simulink model "Helicoptero_2DOF_EKFv2"  (R2024b)
settings: Solver=FixedStepAuto  StartTime=0.0  StopTime=10  FixedStep=0.001  RelTol=1e-3
values from neighbouring files (symbols this model uses):
  theta_0 = -40.5*pi/180    (= -0.706858347058)    [setup_heli_2d_base.m]
  VMAX_UPM_P = 24    [setup_heli_2d_base.m]
  VMAX_UPM_Y = 15    [setup_heli_2d_base.m]
undefined symbols (not defined in the file or in its folder): B_p, B_y, g, J_eq_p, J_eq_y, K_pp, K_py, K_yp, K_yy, l_cm, m_heli
libraries: simulink x3
settings Model: Creator=david  LastModifiedBy=Usuario

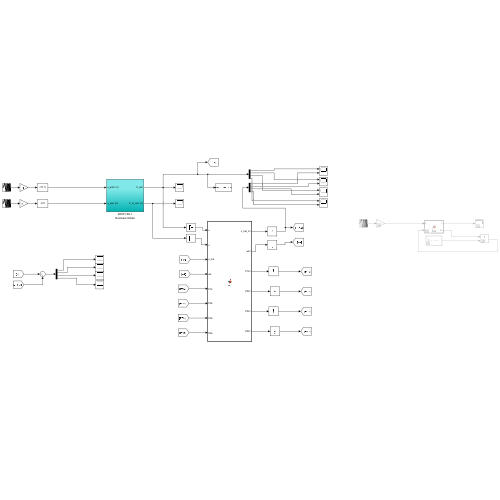
[thumbnail: Simulink's stored preview of the top-level diagram]
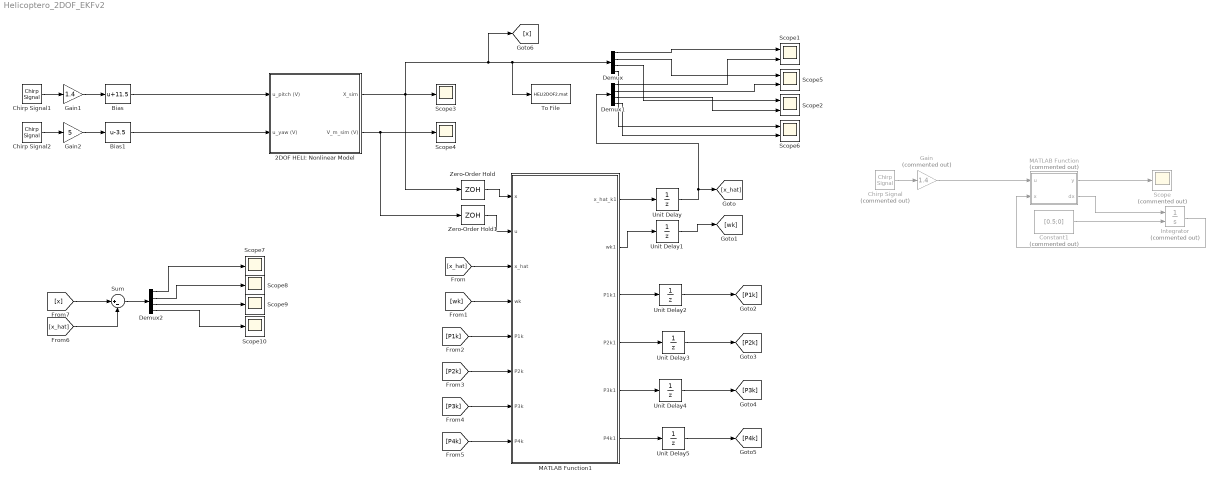
== system Helicoptero_2DOF_EKFv2 ==
  2DOF HELI: Nonlinear Model : Subsystem
  Bias : Bias  Bias=11.5  SaturateOnIntegerOverflow=off
  Bias1 : Bias  Bias=-3.5  SaturateOnIntegerOverflow=off
  Chirp Signal : simulink/Sources/Chirp Signal  Commented=on  f1=0.08  T=10  f2=1
  Chirp Signal1 : simulink/Sources/Chirp Signal  f1=0.08  T=10  f2=1
  Chirp Signal2 : simulink/Sources/Chirp Signal  f1=0.05  T=100  f2=1
  Constant1 : Constant  Commented=on  Value=[0.5;0]
  Demux : Demux
  Demux1 : Demux
  Demux2 : Demux
  Gain : Gain  Commented=on  Gain=1.4
  Gain1 : Gain  Gain=1.4
  Gain2 : Gain  Gain=5
  Integrator : Integrator  Commented=on  InitialConditionSource=external
  MATLAB Function : MATLAB Function  Commented=on  TreatAsAtomicUnit=on
  MATLAB Function1 : MATLAB Function  TreatAsAtomicUnit=on
  Scope : Scope  Commented=on
  Scope{1..2,5..6} (4 alike) : Scope  NumInputPorts=2
  Scope{3..4,7..10} (6 alike) : Scope
  Sum : Sum  Inputs=|+-
  To File : ToFile  Filename=HELI2DOF2.mat  MatrixName=out
  Unit Delay : UnitDelay  SampleTime=-1  HasFrameUpgradeWarning=on
  Unit Delay1 : UnitDelay  InitialCondition=[rand(1,8)]  SampleTime=-1  HasFrameUpgradeWarning=on
  Unit Delay{2..5} (4 alike) : UnitDelay  InitialCondition=eye(2)*50000  SampleTime=-1  HasFrameUpgradeWarning=on
  Zero-Order Hold : ZeroOrderHold  SampleTime=-1
  Zero-Order Hold1 : ZeroOrderHold  SampleTime=-1
  wires:
  MATLAB Function/2(dx) -> Integrator/1
  Integrator/1 -> MATLAB Function/2(x)
  Constant1/1 -> Integrator/2
  MATLAB Function/1(y) -> Scope/1
  Chirp Signal/1 -> Gain/1
  Gain/1 -> MATLAB Function/1(u)
  [P2k] -> MATLAB Function1/6(P2k)
  [P1k] -> MATLAB Function1/5(P1k)
  [wk] -> MATLAB Function1/4(wk)
  [x_hat] -> MATLAB Function1/3(x_hat)
  Demux/1 -> Scope1/1
  Demux/2 -> Scope5/1
  Demux1/1 -> Scope1/2
  Demux1/2 -> Scope5/2
  Unit Delay/1 -> Demux1/1, [x_hat]
  Unit Delay1/1 -> [wk]
  Unit Delay2/1 -> [P1k]
  Unit Delay3/1 -> [P2k]
  MATLAB Function1/1(x_hat_k1) -> Unit Delay/1
  MATLAB Function1/4(P2k1) -> Unit Delay3/1
  MATLAB Function1/3(P1k1) -> Unit Delay2/1
  MATLAB Function1/2(wk1) -> Unit Delay1/1
  Zero-Order Hold/1 -> MATLAB Function1/1(x)
  Zero-Order Hold1/1 -> MATLAB Function1/2(u)
  [P4k] -> MATLAB Function1/8(P4k)
  [P3k] -> MATLAB Function1/7(P3k)
  MATLAB Function1/5(P3k1) -> Unit Delay4/1
  Unit Delay4/1 -> [P3k]
  Unit Delay5/1 -> [P4k]
  MATLAB Function1/6(P4k1) -> Unit Delay5/1
  Gain1/1 -> Bias/1
  Chirp Signal2/1 -> Gain2/1
  Bias1/1 -> 2DOF HELI: Nonlinear Model/2(u_yaw (V))
  Chirp Signal1/1 -> Gain1/1
  Gain2/1 -> Bias1/1
  2DOF HELI: Nonlinear Model/2(V_m_sim (V)) -> Zero-Order Hold1/1, Scope4/1
  Bias/1 -> 2DOF HELI: Nonlinear Model/1(u_pitch (V))
  2DOF HELI: Nonlinear Model/1(X_sim) -> [x], To File/1, Demux/1, Zero-Order Hold/1, Scope3/1
  Demux/3 -> Scope2/1
  Demux1/3 -> Scope2/2
  Demux/4 -> Scope6/1
  Demux1/4 -> Scope6/2
  [x] -> Sum/1
  [x_hat] -> Sum/2
  Sum/1 -> Demux2/1
  Demux2/1 -> Scope7/1
  Demux2/2 -> Scope8/1
  Demux2/3 -> Scope9/1
  Demux2/4 -> Scope10/1

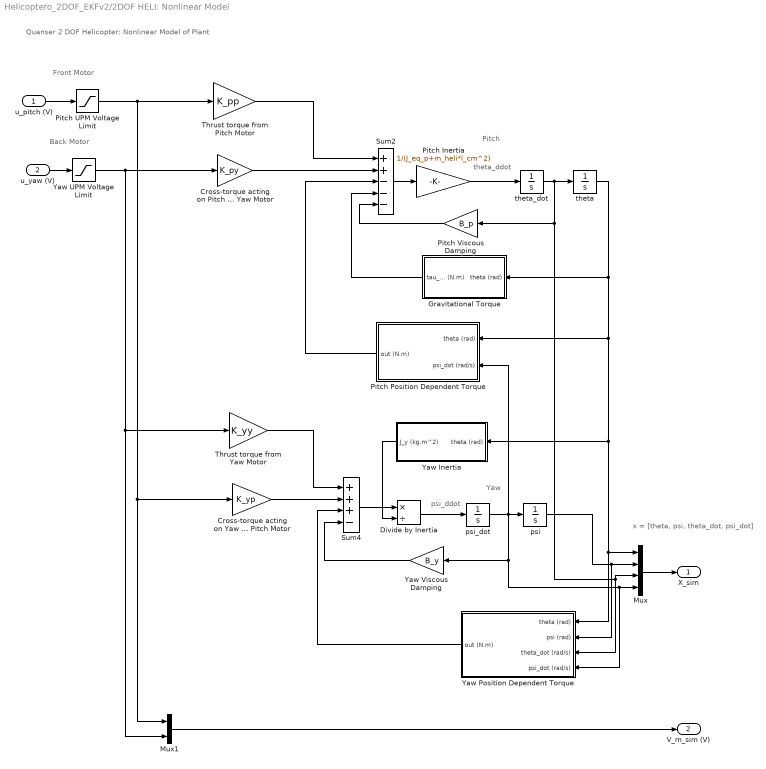
== system Helicoptero_2DOF_EKFv2/2DOF HELI: Nonlinear Model ==
  note: Back Motor
  note: Front Motor
  note: x = [theta, psi, theta_dot, psi_dot]
  note: Quanser 2 DOF Helicopter: Nonlinear Model of Plant
  note: theta_ddot
  note: psi_ddot
  note: Pitch
  note: Yaw
  u_pitch (V) : Inport
  u_yaw (V) : Inport  Port=2
  Cross-torque acting on Pitch from Yaw Motor : Gain  Gain=K_py
  Cross-torque acting on Yaw from Pitch Motor : Gain  Gain=K_yp
  Divide by Inertia : Product  Inputs=*/
  Gravitational Torque : Subsystem
  Mux : Mux
  Mux1 : Mux  Inputs=2
  Pitch Inertia : Gain  Gain=1/(J_eq_p+m_heli*l_cm^2)
  Pitch Position Dependent Torque : Subsystem  AncestorBlock=heli_2d_lib/2DOF Helicopter: Nonlinear Model/Yaw Nonlinear Element
  Pitch UPM Voltage Limit : Saturate  UpperLimit=VMAX_UPM_P  LowerLimit=- VMAX_UPM_P
  Pitch Viscous Damping : Gain  Gain=B_p
  Sum2 : Sum  Inputs=++---
  Sum4 : Sum  Inputs=+++-
  Thrust torque from Pitch Motor : Gain  Gain=K_pp
  Thrust torque from Yaw Motor : Gain  Gain=K_yy
  Yaw Inertia : Subsystem
  Yaw Position Dependent Torque : Subsystem
  Yaw UPM Voltage Limit : Saturate  UpperLimit=VMAX_UPM_Y  LowerLimit=- VMAX_UPM_Y
  Yaw Viscous Damping : Gain  Gain=B_y
  psi : Integrator
  psi_dot : Integrator
  theta : Integrator  InitialCondition=theta_0  LimitOutput=on  UpperSaturationLimit=40.5*pi/180  LowerSaturationLimit=-40.5*pi/180
  theta_dot : Integrator
  X_sim : Outport
  V_m_sim (V) : Outport  Port=2
  wires:
  Pitch Position Dependent Torque/1(out (N.m)) -> Sum2/3
  Gravitational Torque/1(tau_g (N.m)) -> Sum2/4
  Pitch Viscous Damping/1 -> Sum2/5
  Cross-torque acting on Pitch from Yaw Motor/1 -> Sum2/2
  Thrust torque from Pitch Motor/1 -> Sum2/1
  Yaw Inertia/1(J_y (kg.m^2)) -> Divide by Inertia/2
  Divide by Inertia/1 -> psi_dot/1
  Sum4/1 -> Divide by Inertia/1
  Yaw Position Dependent Torque/1(out (N.m)) -> Sum4/3
  Yaw Viscous Damping/1 -> Sum4/4
  psi/1 -> Yaw Position Dependent Torque/2(psi (rad)), Mux/2
  Mux1/1 -> V_m_sim (V)/1
  Yaw UPM Voltage Limit/1 -> Thrust torque from Yaw Motor/1, Mux1/2, Cross-torque acting on Pitch from Yaw Motor/1
  Pitch UPM Voltage Limit/1 -> Mux1/1, Cross-torque acting on Yaw from Pitch Motor/1, Thrust torque from Pitch Motor/1
  Mux/1 -> X_sim/1
  theta/1 -> Gravitational Torque/1(theta (rad)), Pitch Position Dependent Torque/1(theta (rad)), Yaw Position Dependent Torque/1(theta (rad)), Mux/1, Yaw Inertia/1(theta (rad))
  Sum2/1 -> Pitch Inertia/1
  Pitch Inertia/1 -> theta_dot/1
  theta_dot/1 -> Pitch Viscous Damping/1, Yaw Position Dependent Torque/3(theta_dot (rad/s)), Mux/3, theta/1
  Thrust torque from Yaw Motor/1 -> Sum4/1
  Cross-torque acting on Yaw from Pitch Motor/1 -> Sum4/2
  psi_dot/1 -> Yaw Viscous Damping/1, Yaw Position Dependent Torque/4(psi_dot (rad/s)), Mux/4, Pitch Position Dependent Torque/2(psi_dot (rad/s)), psi/1
  u_pitch (V)/1 -> Pitch UPM Voltage Limit/1
  u_yaw (V)/1 -> Yaw UPM Voltage Limit/1

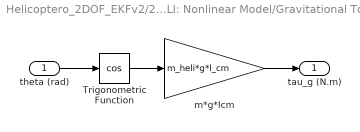
== system Helicoptero_2DOF_EKFv2/2DOF HELI: Nonlinear Model/Gravitational Torque ==
  theta (rad) : Inport
  Trigonometric Function : Trigonometry  Operator=cos  OutputSignalType=real
  m*g*lcm : Gain  Gain=m_heli*g*l_cm
  tau_g (N.m) : Outport
  wires:
  m*g*lcm/1 -> tau_g (N.m)/1
  theta (rad)/1 -> Trigonometric Function/1
  Trigonometric Function/1 -> m*g*lcm/1

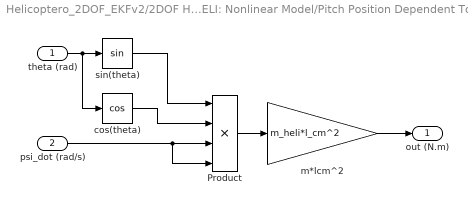
== system Helicoptero_2DOF_EKFv2/2DOF HELI: Nonlinear Model/Pitch Position Dependent Torque ==
  theta (rad) : Inport
  psi_dot (rad/s) : Inport  Port=2
  Product : Product  Inputs=4  RndMeth=Zero
  cos(theta) : Trigonometry  Operator=cos  OutputSignalType=real
  m*lcm^2 : Gain  Gain=m_heli*l_cm^2
  sin(theta) : Trigonometry  OutputSignalType=real
  out (N.m) : Outport
  wires:
  psi_dot (rad/s)/1 -> Product/4, Product/3
  theta (rad)/1 -> cos(theta)/1, sin(theta)/1
  Product/1 -> m*lcm^2/1
  sin(theta)/1 -> Product/1
  cos(theta)/1 -> Product/2
  m*lcm^2/1 -> out (N.m)/1

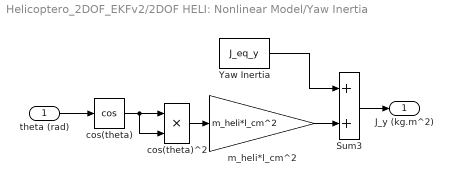
== system Helicoptero_2DOF_EKFv2/2DOF HELI: Nonlinear Model/Yaw Inertia ==
  theta (rad) : Inport
  Sum3 : Sum
  Yaw Inertia : Constant  Value=J_eq_y
  cos(theta) : Trigonometry  Operator=cos  OutputSignalType=real
  cos(theta)^2 : Product  RndMeth=Zero
  m_heli*l_cm^2 : Gain  Gain=m_heli*l_cm^2
  J_y (kg.m^2) : Outport
  wires:
  cos(theta)/1 -> cos(theta)^2/2, cos(theta)^2/1
  Sum3/1 -> J_y (kg.m^2)/1
  theta (rad)/1 -> cos(theta)/1
  m_heli*l_cm^2/1 -> Sum3/2
  Yaw Inertia/1 -> Sum3/1
  cos(theta)^2/1 -> m_heli*l_cm^2/1

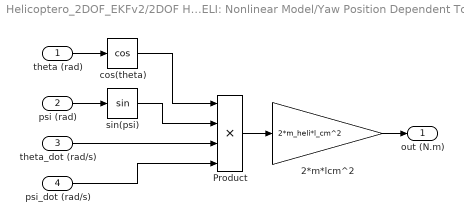
== system Helicoptero_2DOF_EKFv2/2DOF HELI: Nonlinear Model/Yaw Position Dependent Torque ==
  theta (rad) : Inport
  psi (rad) : Inport  Port=2
  theta_dot (rad/s) : Inport  Port=3
  psi_dot (rad/s) : Inport  Port=4
  2*m*lcm^2 : Gain  Gain=2*m_heli*l_cm^2
  Product : Product  Inputs=4  RndMeth=Zero
  cos(theta) : Trigonometry  Operator=cos  OutputSignalType=real
  sin(psi) : Trigonometry  OutputSignalType=real
  out (N.m) : Outport
  wires:
  2*m*lcm^2/1 -> out (N.m)/1
  psi_dot (rad/s)/1 -> Product/4
  theta_dot (rad/s)/1 -> Product/3
  sin(psi)/1 -> Product/2
  cos(theta)/1 -> Product/1
  Product/1 -> 2*m*lcm^2/1
  theta (rad)/1 -> cos(theta)/1
  psi (rad)/1 -> sin(psi)/1

== matlab function Helicoptero_2DOF_EKFv2/MATLAB Function1 ==
  data: x input; u input; x_hat_k1 output; wk1 output; P1k1 output; x_hat input; wk input; P1k input; P2k input; P2k1 output; P3k input; P4k input; P3k1 output; P4k1 output
function [x_hat_k1,wk1,P1k1,P2k1,P3k1,P4k1] = fcn(x,u,x_hat,wk,P1k,P2k,P3k,P4k)

%% Constant weights

w_1=0.15;
%w_2=0.1; %Revisar que valores podemos usar


%% Neural states

x_hat_k_1 = wk(1)*tanh(x(3)) +  wk(2)*tanh(x(1));
x_hat_k_2 = wk(3)*tanh(x(4)) +  wk(4)*tanh(x(2));

x_hat_k_3 = wk(5)*tanh(x(3)) +  wk(6)*tanh(x(1))*cos(x(1))^2 + w_1*u(1);
x_hat_k_4 = wk(7)*tanh(x(4)) +  wk(8)*tanh(x(2))*cos(x(2)) + w_1*u(2);


x_hat_k1 = [x_hat_k_1;x_hat_k_2;x_hat_k_3;x_hat_k_4];


%% H matrix coeff

H1=[tanh(x(3)) tanh(x(1))]';
H2=[tanh(x(4)) tanh(x(2))]';
H3=[tanh(x(3)) tanh(x(1))*cos(x(1))^2]';
H4=[tanh(x(4)) tanh(x(2))*cos(x(2))]';



%% EKF computation per each state

Q1=eye(2)*5e3;
R1=6e3;

Q2=Q1;
R2=R1;

Q3=Q1;
R3=R1;

Q4=Q1;
R4=R1;



%error
error=x-x_hat;


% First filter

K1=(P1k*H1)/(R1+H1'*P1k*H1);
w1k1=[wk(1);wk(2)]+K1*error(1);
P1k1=P1k-K1*H1'*P1k+Q1;


% Second filter


K2=P2k*H2/(R2+H2'*P2k*H2);
w2k1=[wk(3);wk(4)]+K2*error(2);
P2k1=P2k-K2*H2'*P2k+Q2;


% Third filter

K3=(P3k*H3)/(R3+H3'*P3k*H3);
w3k1=[wk(5);wk(6)]+K3*error(3);
P3k1=P3k-K3*H3'*P3k+Q3;


% Fourth filter

K4=(P4k*H4)/(R4+H4'*P4k*H4);
w4k1=[wk(7);wk(8)]+K4*error(4);
P4k1=P4k-K4*H4'*P4k+Q4;



wk1=[w1k1;w2k1;w3k1;w4k1];

== matlab function Helicoptero_2DOF_EKFv2/MATLAB Function ==
  data: y output; dx output; u input; x input
function [y, dx] = fcn(u, x)
g = 9.81;  
l = 1;     
m = 1;     
b = 0.5;   

x1 = x(1);  
x2 = x(2);  

dx1 = x2;
dx2 = -(g/l)*sin(x1) - (b*l/(m*l^2))*x2 + u/(m*l^2);

dx = [dx1; dx2];

y = x1;
